simulink library "csu_tcm_thruster_command_metering_lib"  (R2014b)
settings: Solver=ode45  StartTime=0.0  StopTime=10.0  RelTol=1e-3
values from neighbouring files (symbols this model uses):
  act_full_on_duration = uint32( 120 )    [csc_act_actuator_manager_init.m]
libraries: util_common_lib x4, simulink x1, util_info_lib x1
settings Model: Creator=escrane  LastModifiedBy=mstewart

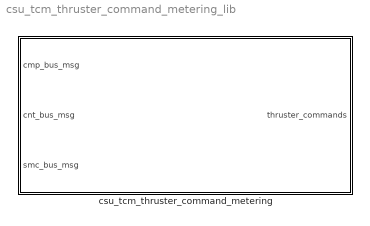
== system csu_tcm_thruster_command_metering_lib ==
  csu_tcm_thruster_command_metering : Subsystem

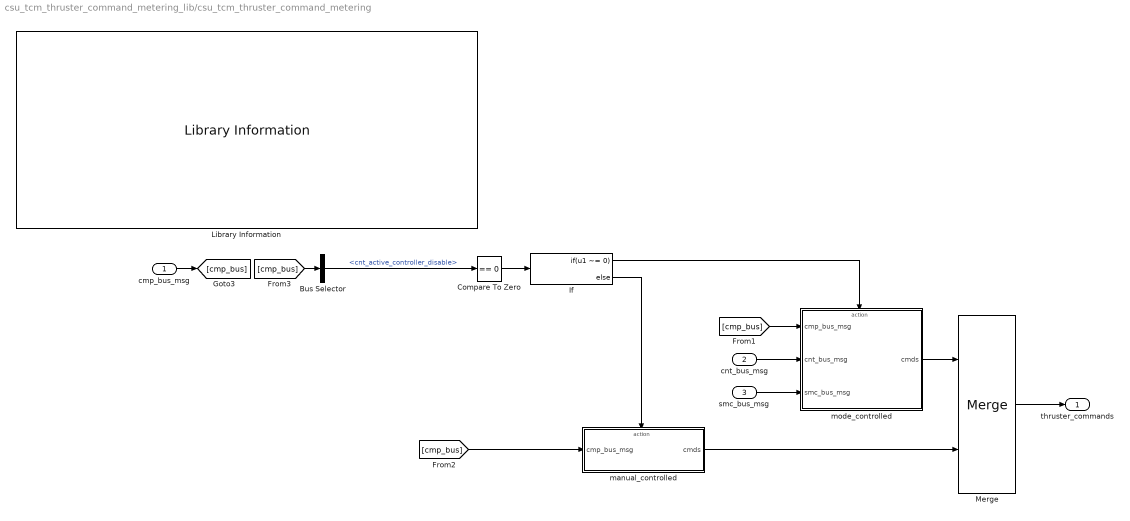
== system csu_tcm_thruster_command_metering_lib/csu_tcm_thruster_command_metering ==
  cmp_bus_msg : Inport
  cnt_bus_msg : Inport  Port=2
  smc_bus_msg : Inport  Port=3
  Bus Selector : BusSelector  OutputSignals=cnt_active_controller_disable
  Compare To Zero : simulink/Logic and Bit Operations/Compare To Zero  relop===  OutDataTypeStr=boolean
  If : If  IfExpression=u1 ~= 0
  Library Information : util_info_lib/Library Information  owner='escrane'
  Merge : Merge
  manual_controlled : Subsystem  TreatAsAtomicUnit=on
  mode_controlled : Subsystem  TreatAsAtomicUnit=on
  thruster_commands : Outport
  wires:
  [cmp_bus] -> manual_controlled/1(cmp_bus_msg)
  If/2 -> manual_controlled/Action
  If/1 -> mode_controlled/Action
  Compare To Zero/1 -> If/1
  [cmp_bus] -> mode_controlled/1(cmp_bus_msg)
  cnt_bus_msg/1 -> mode_controlled/2(cnt_bus_msg)
  smc_bus_msg/1 -> mode_controlled/3(smc_bus_msg)
  [cmp_bus] -> Bus Selector/1
  cmp_bus_msg/1 -> [cmp_bus]
  Merge/1 -> thruster_commands/1
  manual_controlled/1(cmds) -> Merge/2
  mode_controlled/1(cmds) -> Merge/1
  Bus Selector/1 -> Compare To Zero/1  "<cnt_active_controller_disable>"

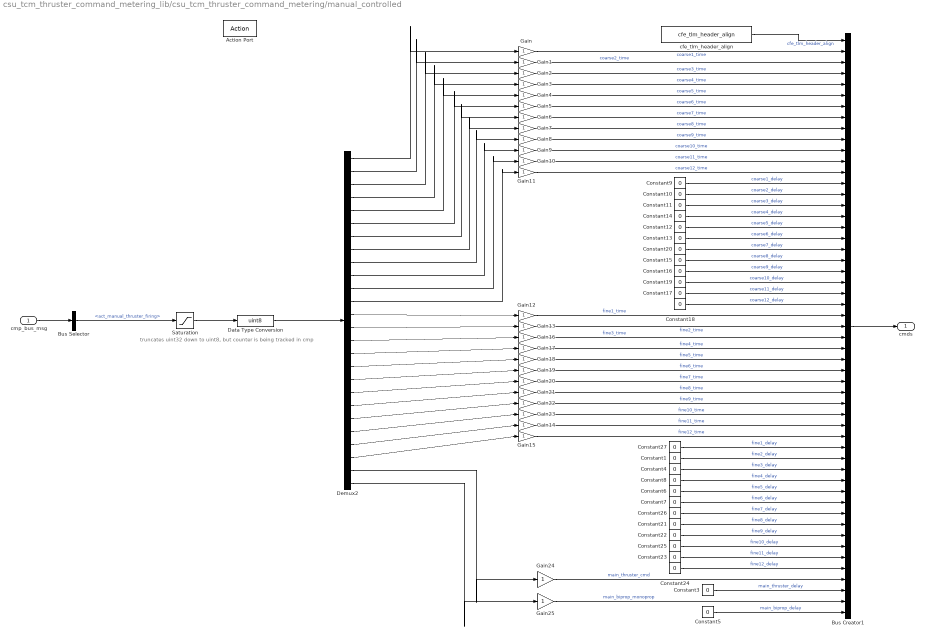
== system csu_tcm_thruster_command_metering_lib/csu_tcm_thruster_command_metering/manual_controlled ==
  note: truncates uint32 down to uint8, but counter is being tracked in cmp
  cmp_bus_msg : Inport
  Action Port : ActionPort
  Bus Creator1 : BusCreator  Inputs=53
  Bus Selector : BusSelector  OutputSignals=act_manual_thruster_firing
  Constant{1,3..27} (26 alike) : Constant  Value=0  OutDataTypeStr=uint8
  Data Type Conversion : DataTypeConversion  OutDataTypeStr=uint8
  Demux2 : Demux  Outputs=26
  Gain{,1..25} (26 alike) : Gain  OutDataTypeStr=uint8
  Saturation : Saturate  UpperLimit=act_full_on_duration  LowerLimit=0
  cfe_tlm_header_align : util_common_lib/cfe_tlm_header_align
  cmds : Outport
  wires:
  Data Type Conversion/1 -> Demux2/1
  Demux2/24 -> Gain15/1
  Demux2/23 -> Gain14/1
  Demux2/22 -> Gain23/1
  Demux2/21 -> Gain22/1
  Demux2/20 -> Gain21/1
  Demux2/19 -> Gain20/1
  Demux2/18 -> Gain19/1
  Demux2/17 -> Gain18/1
  Demux2/16 -> Gain17/1
  Demux2/15 -> Gain16/1
  Demux2/13 -> Gain12/1
  Gain18/1 -> Bus Creator1/30  "fine5_time"
  Gain17/1 -> Bus Creator1/29  "fine4_time"
  Gain13/1 -> Bus Creator1/27  "fine2_time"
  Gain16/1 -> Bus Creator1/28  "fine3_time"
  Demux2/1 -> Gain/1
  Demux2/2 -> Gain1/1
  Demux2/3 -> Gain2/1
  Demux2/4 -> Gain3/1
  Demux2/5 -> Gain4/1
  Demux2/6 -> Gain5/1
  Demux2/12 -> Gain11/1
  Demux2/11 -> Gain10/1
  Demux2/10 -> Gain9/1
  Demux2/9 -> Gain8/1
  Demux2/26 -> Gain25/1
  Demux2/25 -> Gain24/1
  Demux2/8 -> Gain7/1
  Demux2/7 -> Gain6/1
  Bus Selector/1 -> Saturation/1  "<act_manual_thruster_firing>"
  cmp_bus_msg/1 -> Bus Selector/1
  Gain25/1 -> Bus Creator1/52  "main_biprop_monoprop"
  Gain24/1 -> Bus Creator1/50  "main_thruster_cmd"
  Gain3/1 -> Bus Creator1/5  "coarse4_time"
  Bus Creator1/1 -> cmds/1
  cfe_tlm_header_align/1 -> Bus Creator1/1  "cfe_tlm_header_align"
  Gain/1 -> Bus Creator1/2  "coarse1_time"
  Gain7/1 -> Bus Creator1/9  "coarse8_time"
  Gain8/1 -> Bus Creator1/10  "coarse9_time"
  Gain11/1 -> Bus Creator1/13  "coarse12_time"
  Gain6/1 -> Bus Creator1/8  "coarse7_time"
  Gain5/1 -> Bus Creator1/7  "coarse6_time"
  Gain2/1 -> Bus Creator1/4  "coarse3_time"
  Gain4/1 -> Bus Creator1/6  "coarse5_time"
  Gain9/1 -> Bus Creator1/11  "coarse10_time"
  Gain1/1 -> Bus Creator1/3  "coarse2_time"
  Gain10/1 -> Bus Creator1/12  "coarse11_time"
  Constant11/1 -> Bus Creator1/16  "coarse3_delay"
  Constant14/1 -> Bus Creator1/17  "coarse4_delay"
  Constant13/1 -> Bus Creator1/19  "coarse6_delay"
  Constant15/1 -> Bus Creator1/21  "coarse8_delay"
  Constant10/1 -> Bus Creator1/15  "coarse2_delay"
  Constant18/1 -> Bus Creator1/25  "coarse12_delay"
  Constant16/1 -> Bus Creator1/22  "coarse9_delay"
  Constant12/1 -> Bus Creator1/18  "coarse5_delay"
  Constant9/1 -> Bus Creator1/14  "coarse1_delay"
  Constant17/1 -> Bus Creator1/24  "coarse11_delay"
  Constant20/1 -> Bus Creator1/20  "coarse7_delay"
  Constant19/1 -> Bus Creator1/23  "coarse10_delay"
  Gain22/1 -> Bus Creator1/34  "fine9_time"
  Gain23/1 -> Bus Creator1/35  "fine10_time"
  Gain21/1 -> Bus Creator1/33  "fine8_time"
  Gain20/1 -> Bus Creator1/32  "fine7_time"
  Demux2/14 -> Gain13/1
  Gain12/1 -> Bus Creator1/26  "fine1_time"
  Gain15/1 -> Bus Creator1/37  "fine12_time"
  Gain19/1 -> Bus Creator1/31  "fine6_time"
  Gain14/1 -> Bus Creator1/36  "fine11_time"
  Constant5/1 -> Bus Creator1/53  "main_biprop_delay"
  Constant3/1 -> Bus Creator1/51  "main_thruster_delay"
  Constant27/1 -> Bus Creator1/38  "fine1_delay"
  Constant25/1 -> Bus Creator1/47  "fine10_delay"
  Constant8/1 -> Bus Creator1/41  "fine4_delay"
  Constant22/1 -> Bus Creator1/46  "fine9_delay"
  Constant7/1 -> Bus Creator1/43  "fine6_delay"
  Constant4/1 -> Bus Creator1/40  "fine3_delay"
  Constant21/1 -> Bus Creator1/45  "fine8_delay"
  Constant6/1 -> Bus Creator1/42  "fine5_delay"
  Constant1/1 -> Bus Creator1/39  "fine2_delay"
  Constant24/1 -> Bus Creator1/49  "fine12_delay"
  Constant26/1 -> Bus Creator1/44  "fine7_delay"
  Constant23/1 -> Bus Creator1/48  "fine11_delay"
  Saturation/1 -> Data Type Conversion/1

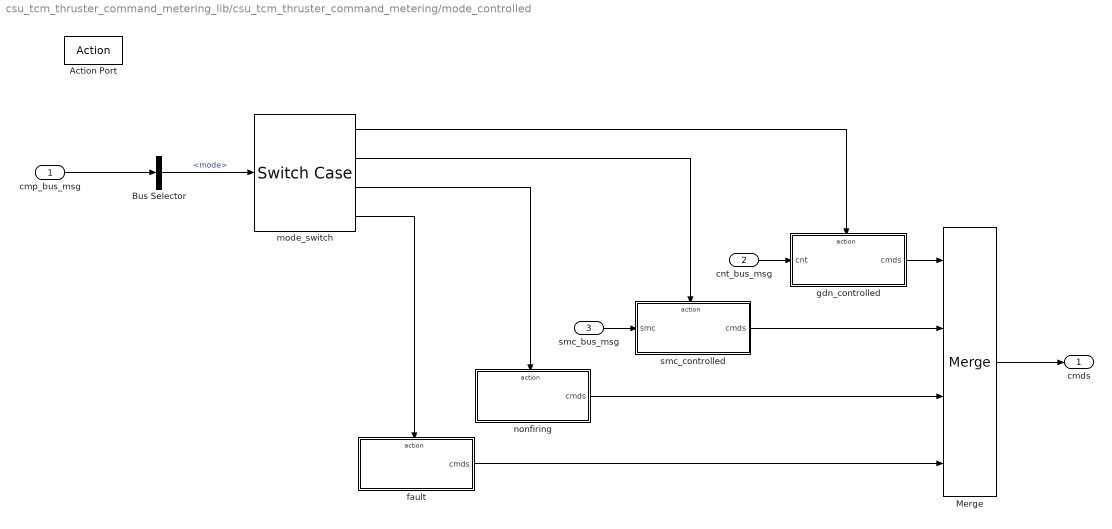
== system csu_tcm_thruster_command_metering_lib/csu_tcm_thruster_command_metering/mode_controlled ==
  cmp_bus_msg : Inport
  cnt_bus_msg : Inport  Port=2
  smc_bus_msg : Inport  Port=3
  Action Port : ActionPort
  Bus Selector : BusSelector  OutputSignals=mode
  Merge : Merge  Inputs=4
  fault : Subsystem  TreatAsAtomicUnit=on
  gdn_controlled : Subsystem  TreatAsAtomicUnit=on
  mode_switch : SwitchCase  CaseConditions={ [uint8(enum_mode.pointing), uint8(enum_mode.deltav), uint8(enum_mode.deorbit), uint8(enum_mode.braking) uint8(enum_mode.landing)], uint8(enum_mode.safe), [uint8(enum_mode.startup), uint8(enum_mode.surface), uint8(enum_mode.safesurface)]}
  nonfiring : Subsystem  TreatAsAtomicUnit=on
  smc_controlled : Subsystem  TreatAsAtomicUnit=on
  cmds : Outport
  wires:
  cmp_bus_msg/1 -> Bus Selector/1
  fault/1(cmds) -> Merge/4
  mode_switch/4 -> fault/Action
  Merge/1 -> cmds/1
  smc_bus_msg/1 -> smc_controlled/1(smc)
  nonfiring/1(cmds) -> Merge/3
  smc_controlled/1(cmds) -> Merge/2
  gdn_controlled/1(cmds) -> Merge/1
  mode_switch/3 -> nonfiring/Action
  mode_switch/2 -> smc_controlled/Action
  mode_switch/1 -> gdn_controlled/Action
  cnt_bus_msg/1 -> gdn_controlled/1(cnt)
  Bus Selector/1 -> mode_switch/1  "<mode>"

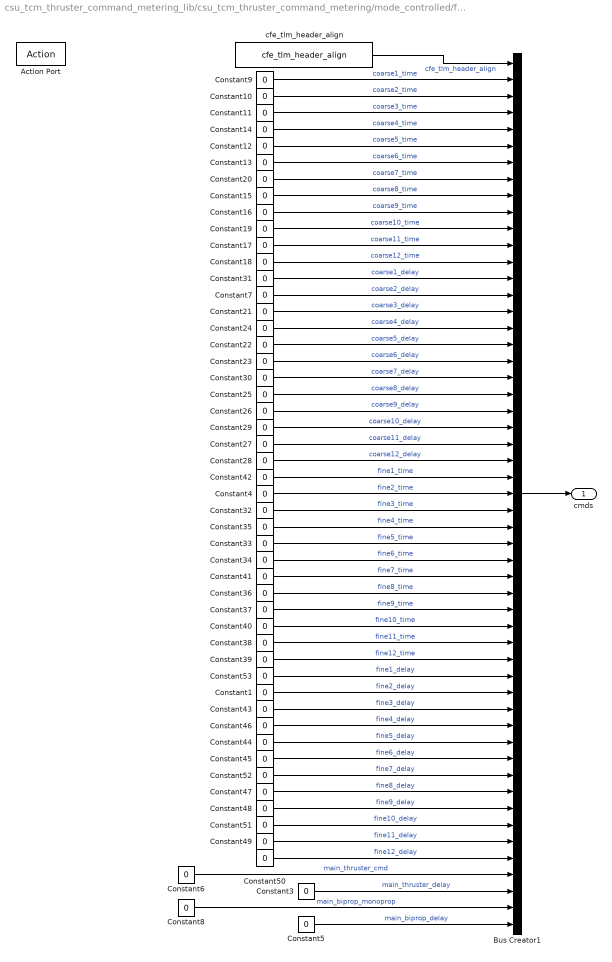
== system csu_tcm_thruster_command_metering_lib/csu_tcm_thruster_command_metering/mode_controlled/fault ==
  Action Port : ActionPort
  Bus Creator1 : BusCreator  Inputs=53
  Constant{1,3..53} (52 alike) : Constant  Value=0  OutDataTypeStr=uint8
  cfe_tlm_header_align : util_common_lib/cfe_tlm_header_align
  cmds : Outport
  wires:
  Bus Creator1/1 -> cmds/1
  Constant8/1 -> Bus Creator1/52  "main_biprop_monoprop"
  Constant6/1 -> Bus Creator1/50  "main_thruster_cmd"
  cfe_tlm_header_align/1 -> Bus Creator1/1  "cfe_tlm_header_align"
  Constant9/1 -> Bus Creator1/2  "coarse1_time"
  Constant15/1 -> Bus Creator1/9  "coarse8_time"
  Constant16/1 -> Bus Creator1/10  "coarse9_time"
  Constant18/1 -> Bus Creator1/13  "coarse12_time"
  Constant20/1 -> Bus Creator1/8  "coarse7_time"
  Constant14/1 -> Bus Creator1/5  "coarse4_time"
  Constant13/1 -> Bus Creator1/7  "coarse6_time"
  Constant11/1 -> Bus Creator1/4  "coarse3_time"
  Constant12/1 -> Bus Creator1/6  "coarse5_time"
  Constant19/1 -> Bus Creator1/11  "coarse10_time"
  Constant10/1 -> Bus Creator1/3  "coarse2_time"
  Constant17/1 -> Bus Creator1/12  "coarse11_time"
  Constant21/1 -> Bus Creator1/16  "coarse3_delay"
  Constant24/1 -> Bus Creator1/17  "coarse4_delay"
  Constant23/1 -> Bus Creator1/19  "coarse6_delay"
  Constant25/1 -> Bus Creator1/21  "coarse8_delay"
  Constant7/1 -> Bus Creator1/15  "coarse2_delay"
  Constant28/1 -> Bus Creator1/25  "coarse12_delay"
  Constant26/1 -> Bus Creator1/22  "coarse9_delay"
  Constant22/1 -> Bus Creator1/18  "coarse5_delay"
  Constant31/1 -> Bus Creator1/14  "coarse1_delay"
  Constant27/1 -> Bus Creator1/24  "coarse11_delay"
  Constant30/1 -> Bus Creator1/20  "coarse7_delay"
  Constant29/1 -> Bus Creator1/23  "coarse10_delay"
  Constant35/1 -> Bus Creator1/29  "fine4_time"
  Constant37/1 -> Bus Creator1/34  "fine9_time"
  Constant40/1 -> Bus Creator1/35  "fine10_time"
  Constant36/1 -> Bus Creator1/33  "fine8_time"
  Constant41/1 -> Bus Creator1/32  "fine7_time"
  Constant4/1 -> Bus Creator1/27  "fine2_time"
  Constant42/1 -> Bus Creator1/26  "fine1_time"
  Constant33/1 -> Bus Creator1/30  "fine5_time"
  Constant39/1 -> Bus Creator1/37  "fine12_time"
  Constant32/1 -> Bus Creator1/28  "fine3_time"
  Constant34/1 -> Bus Creator1/31  "fine6_time"
  Constant38/1 -> Bus Creator1/36  "fine11_time"
  Constant5/1 -> Bus Creator1/53  "main_biprop_delay"
  Constant3/1 -> Bus Creator1/51  "main_thruster_delay"
  Constant53/1 -> Bus Creator1/38  "fine1_delay"
  Constant51/1 -> Bus Creator1/47  "fine10_delay"
  Constant46/1 -> Bus Creator1/41  "fine4_delay"
  Constant48/1 -> Bus Creator1/46  "fine9_delay"
  Constant45/1 -> Bus Creator1/43  "fine6_delay"
  Constant43/1 -> Bus Creator1/40  "fine3_delay"
  Constant47/1 -> Bus Creator1/45  "fine8_delay"
  Constant44/1 -> Bus Creator1/42  "fine5_delay"
  Constant1/1 -> Bus Creator1/39  "fine2_delay"
  Constant50/1 -> Bus Creator1/49  "fine12_delay"
  Constant52/1 -> Bus Creator1/44  "fine7_delay"
  Constant49/1 -> Bus Creator1/48  "fine11_delay"

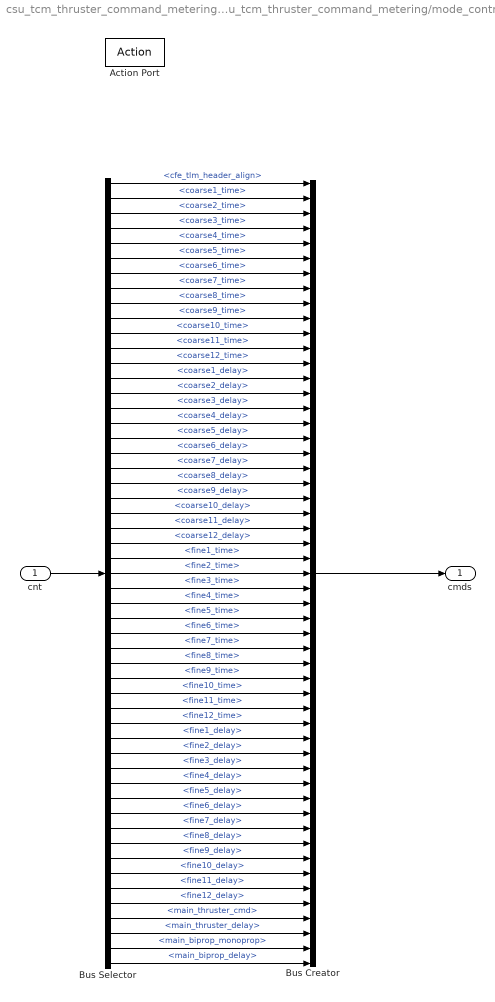
== system csu_tcm_thruster_command_metering_lib/csu_tcm_thruster_command_metering/mode_controlled/gdn_controlled ==
  cnt : Inport
  Action Port : ActionPort
  Bus Creator : BusCreator  Inputs=53
  Bus Selector : BusSelector  OutputSignals=cfe_tlm_header_align,coarse1_time,coarse2_time,coarse3_time,coarse4_time,coarse5_time,coarse6_time,coarse7_time,coarse8_time,coarse9_time,coarse10_time,coarse11_time,coarse12_time,coarse1_delay,coarse2_delay,coarse3_delay,coarse4_delay,coarse5_delay,coarse6_delay,coarse7_delay,coarse8_delay,coarse9_delay,coarse10_delay,coarse11_delay,coarse12_delay,fine1_time,fine2_time,fine3_time,fine4_time,fine5_time,fine6_time,fine7_time,fine8_time,fine9_time,fine10_time,fine11_time,fine12_time,fine1_delay,fine2_delay,fine3_delay,fine4_delay,fine5_delay,fine6_delay,fine7_delay,fine8_delay,fine9_delay,fine10_delay,fine11_delay,fine12_delay,main_thruster_cmd,main_thruster_delay,main_biprop_monoprop,main_biprop_delay
  cmds : Outport
  wires:
  Bus Creator/1 -> cmds/1
  Bus Selector/39 -> Bus Creator/39  "<fine2_delay>"
  Bus Selector/3 -> Bus Creator/3  "<coarse2_time>"
  Bus Selector/27 -> Bus Creator/27  "<fine2_time>"
  Bus Selector/7 -> Bus Creator/7  "<coarse6_time>"
  Bus Selector/50 -> Bus Creator/50  "<main_thruster_cmd>"
  Bus Selector/1 -> Bus Creator/1  "<cfe_tlm_header_align>"
  Bus Selector/18 -> Bus Creator/18  "<coarse5_delay>"
  Bus Selector/42 -> Bus Creator/42  "<fine5_delay>"
  Bus Selector/17 -> Bus Creator/17  "<coarse4_delay>"
  Bus Selector/11 -> Bus Creator/11  "<coarse10_time>"
  Bus Selector/40 -> Bus Creator/40  "<fine3_delay>"
  Bus Selector/10 -> Bus Creator/10  "<coarse9_time>"
  Bus Selector/43 -> Bus Creator/43  "<fine6_delay>"
  Bus Selector/9 -> Bus Creator/9  "<coarse8_time>"
  Bus Selector/28 -> Bus Creator/28  "<fine3_time>"
  Bus Selector/35 -> Bus Creator/35  "<fine10_time>"
  Bus Selector/51 -> Bus Creator/51  "<main_thruster_delay>"
  Bus Selector/37 -> Bus Creator/37  "<fine12_time>"
  Bus Selector/13 -> Bus Creator/13  "<coarse12_time>"
  Bus Selector/21 -> Bus Creator/21  "<coarse8_delay>"
  Bus Selector/38 -> Bus Creator/38  "<fine1_delay>"
  Bus Selector/31 -> Bus Creator/31  "<fine6_time>"
  Bus Selector/6 -> Bus Creator/6  "<coarse5_time>"
  Bus Selector/24 -> Bus Creator/24  "<coarse11_delay>"
  Bus Selector/4 -> Bus Creator/4  "<coarse3_time>"
  Bus Selector/12 -> Bus Creator/12  "<coarse11_time>"
  Bus Selector/23 -> Bus Creator/23  "<coarse10_delay>"
  Bus Selector/33 -> Bus Creator/33  "<fine8_time>"
  Bus Selector/22 -> Bus Creator/22  "<coarse9_delay>"
  Bus Selector/44 -> Bus Creator/44  "<fine7_delay>"
  Bus Selector/45 -> Bus Creator/45  "<fine8_delay>"
  Bus Selector/20 -> Bus Creator/20  "<coarse7_delay>"
  Bus Selector/47 -> Bus Creator/47  "<fine10_delay>"
  Bus Selector/16 -> Bus Creator/16  "<coarse3_delay>"
  Bus Selector/53 -> Bus Creator/53  "<main_biprop_delay>"
  Bus Selector/34 -> Bus Creator/34  "<fine9_time>"
  Bus Selector/49 -> Bus Creator/49  "<fine12_delay>"
  Bus Selector/5 -> Bus Creator/5  "<coarse4_time>"
  Bus Selector/26 -> Bus Creator/26  "<fine1_time>"
  Bus Selector/48 -> Bus Creator/48  "<fine11_delay>"
  Bus Selector/8 -> Bus Creator/8  "<coarse7_time>"
  Bus Selector/52 -> Bus Creator/52  "<main_biprop_monoprop>"
  Bus Selector/46 -> Bus Creator/46  "<fine9_delay>"
  Bus Selector/32 -> Bus Creator/32  "<fine7_time>"
  Bus Selector/19 -> Bus Creator/19  "<coarse6_delay>"
  Bus Selector/2 -> Bus Creator/2  "<coarse1_time>"
  Bus Selector/25 -> Bus Creator/25  "<coarse12_delay>"
  Bus Selector/30 -> Bus Creator/30  "<fine5_time>"
  Bus Selector/36 -> Bus Creator/36  "<fine11_time>"
  Bus Selector/14 -> Bus Creator/14  "<coarse1_delay>"
  Bus Selector/41 -> Bus Creator/41  "<fine4_delay>"
  Bus Selector/15 -> Bus Creator/15  "<coarse2_delay>"
  Bus Selector/29 -> Bus Creator/29  "<fine4_time>"
  cnt/1 -> Bus Selector/1

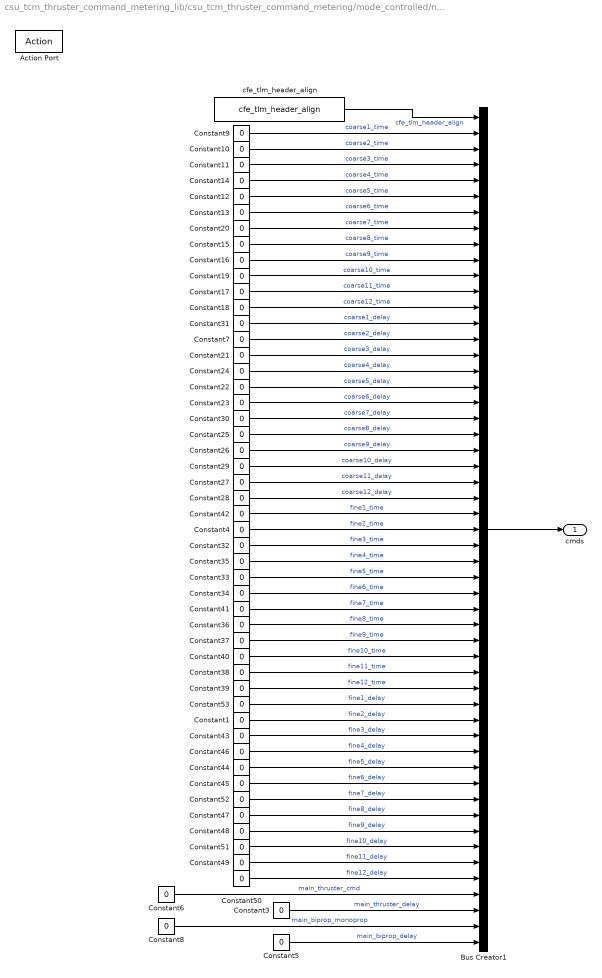
== system csu_tcm_thruster_command_metering_lib/csu_tcm_thruster_command_metering/mode_controlled/nonfiring ==
  Action Port : ActionPort
  Bus Creator1 : BusCreator  Inputs=53
  Constant{1,3..53} (52 alike) : Constant  Value=0  OutDataTypeStr=uint8
  cfe_tlm_header_align : util_common_lib/cfe_tlm_header_align
  cmds : Outport
  wires:
  Constant8/1 -> Bus Creator1/52  "main_biprop_monoprop"
  Constant6/1 -> Bus Creator1/50  "main_thruster_cmd"
  cfe_tlm_header_align/1 -> Bus Creator1/1  "cfe_tlm_header_align"
  Constant9/1 -> Bus Creator1/2  "coarse1_time"
  Constant15/1 -> Bus Creator1/9  "coarse8_time"
  Constant16/1 -> Bus Creator1/10  "coarse9_time"
  Constant18/1 -> Bus Creator1/13  "coarse12_time"
  Constant20/1 -> Bus Creator1/8  "coarse7_time"
  Constant14/1 -> Bus Creator1/5  "coarse4_time"
  Constant13/1 -> Bus Creator1/7  "coarse6_time"
  Constant11/1 -> Bus Creator1/4  "coarse3_time"
  Constant12/1 -> Bus Creator1/6  "coarse5_time"
  Constant19/1 -> Bus Creator1/11  "coarse10_time"
  Constant10/1 -> Bus Creator1/3  "coarse2_time"
  Constant17/1 -> Bus Creator1/12  "coarse11_time"
  Constant21/1 -> Bus Creator1/16  "coarse3_delay"
  Constant24/1 -> Bus Creator1/17  "coarse4_delay"
  Constant23/1 -> Bus Creator1/19  "coarse6_delay"
  Constant25/1 -> Bus Creator1/21  "coarse8_delay"
  Constant7/1 -> Bus Creator1/15  "coarse2_delay"
  Constant28/1 -> Bus Creator1/25  "coarse12_delay"
  Constant26/1 -> Bus Creator1/22  "coarse9_delay"
  Constant22/1 -> Bus Creator1/18  "coarse5_delay"
  Constant31/1 -> Bus Creator1/14  "coarse1_delay"
  Constant27/1 -> Bus Creator1/24  "coarse11_delay"
  Constant30/1 -> Bus Creator1/20  "coarse7_delay"
  Constant29/1 -> Bus Creator1/23  "coarse10_delay"
  Constant35/1 -> Bus Creator1/29  "fine4_time"
  Constant37/1 -> Bus Creator1/34  "fine9_time"
  Constant40/1 -> Bus Creator1/35  "fine10_time"
  Constant36/1 -> Bus Creator1/33  "fine8_time"
  Constant41/1 -> Bus Creator1/32  "fine7_time"
  Constant4/1 -> Bus Creator1/27  "fine2_time"
  Constant42/1 -> Bus Creator1/26  "fine1_time"
  Constant33/1 -> Bus Creator1/30  "fine5_time"
  Constant39/1 -> Bus Creator1/37  "fine12_time"
  Constant32/1 -> Bus Creator1/28  "fine3_time"
  Constant34/1 -> Bus Creator1/31  "fine6_time"
  Constant38/1 -> Bus Creator1/36  "fine11_time"
  Constant5/1 -> Bus Creator1/53  "main_biprop_delay"
  Constant3/1 -> Bus Creator1/51  "main_thruster_delay"
  Constant53/1 -> Bus Creator1/38  "fine1_delay"
  Constant51/1 -> Bus Creator1/47  "fine10_delay"
  Constant46/1 -> Bus Creator1/41  "fine4_delay"
  Constant48/1 -> Bus Creator1/46  "fine9_delay"
  Constant45/1 -> Bus Creator1/43  "fine6_delay"
  Constant43/1 -> Bus Creator1/40  "fine3_delay"
  Constant47/1 -> Bus Creator1/45  "fine8_delay"
  Constant44/1 -> Bus Creator1/42  "fine5_delay"
  Constant1/1 -> Bus Creator1/39  "fine2_delay"
  Constant50/1 -> Bus Creator1/49  "fine12_delay"
  Constant52/1 -> Bus Creator1/44  "fine7_delay"
  Constant49/1 -> Bus Creator1/48  "fine11_delay"
  Bus Creator1/1 -> cmds/1

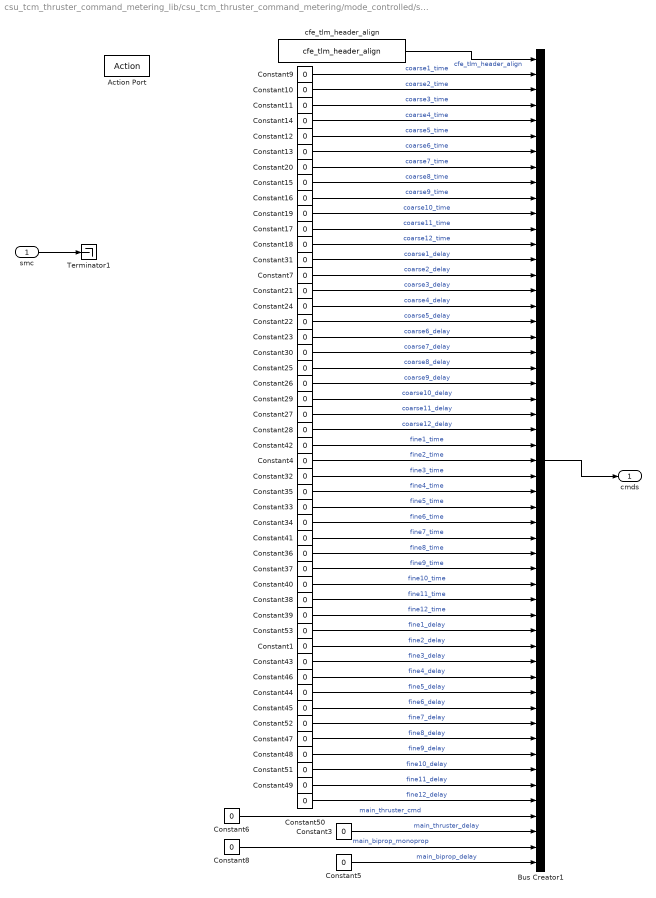
== system csu_tcm_thruster_command_metering_lib/csu_tcm_thruster_command_metering/mode_controlled/smc_controlled ==
  smc : Inport
  Action Port : ActionPort
  Bus Creator1 : BusCreator  Inputs=53
  Constant{1,3..53} (52 alike) : Constant  Value=0  OutDataTypeStr=uint8
  Terminator1 : Terminator
  cfe_tlm_header_align : util_common_lib/cfe_tlm_header_align
  cmds : Outport
  wires:
  Constant8/1 -> Bus Creator1/52  "main_biprop_monoprop"
  Constant6/1 -> Bus Creator1/50  "main_thruster_cmd"
  cfe_tlm_header_align/1 -> Bus Creator1/1  "cfe_tlm_header_align"
  Constant9/1 -> Bus Creator1/2  "coarse1_time"
  Constant15/1 -> Bus Creator1/9  "coarse8_time"
  Constant16/1 -> Bus Creator1/10  "coarse9_time"
  Constant18/1 -> Bus Creator1/13  "coarse12_time"
  Constant20/1 -> Bus Creator1/8  "coarse7_time"
  Constant14/1 -> Bus Creator1/5  "coarse4_time"
  Constant13/1 -> Bus Creator1/7  "coarse6_time"
  Constant11/1 -> Bus Creator1/4  "coarse3_time"
  Constant12/1 -> Bus Creator1/6  "coarse5_time"
  Constant19/1 -> Bus Creator1/11  "coarse10_time"
  Constant10/1 -> Bus Creator1/3  "coarse2_time"
  Constant17/1 -> Bus Creator1/12  "coarse11_time"
  Constant21/1 -> Bus Creator1/16  "coarse3_delay"
  Constant24/1 -> Bus Creator1/17  "coarse4_delay"
  Constant23/1 -> Bus Creator1/19  "coarse6_delay"
  Constant25/1 -> Bus Creator1/21  "coarse8_delay"
  Constant7/1 -> Bus Creator1/15  "coarse2_delay"
  Constant28/1 -> Bus Creator1/25  "coarse12_delay"
  Constant26/1 -> Bus Creator1/22  "coarse9_delay"
  Constant22/1 -> Bus Creator1/18  "coarse5_delay"
  Constant31/1 -> Bus Creator1/14  "coarse1_delay"
  Constant27/1 -> Bus Creator1/24  "coarse11_delay"
  Constant30/1 -> Bus Creator1/20  "coarse7_delay"
  Constant29/1 -> Bus Creator1/23  "coarse10_delay"
  Constant35/1 -> Bus Creator1/29  "fine4_time"
  Constant37/1 -> Bus Creator1/34  "fine9_time"
  Constant40/1 -> Bus Creator1/35  "fine10_time"
  Constant36/1 -> Bus Creator1/33  "fine8_time"
  Constant41/1 -> Bus Creator1/32  "fine7_time"
  Constant4/1 -> Bus Creator1/27  "fine2_time"
  Constant42/1 -> Bus Creator1/26  "fine1_time"
  Constant33/1 -> Bus Creator1/30  "fine5_time"
  Constant39/1 -> Bus Creator1/37  "fine12_time"
  Constant32/1 -> Bus Creator1/28  "fine3_time"
  Constant34/1 -> Bus Creator1/31  "fine6_time"
  Constant38/1 -> Bus Creator1/36  "fine11_time"
  Constant5/1 -> Bus Creator1/53  "main_biprop_delay"
  Constant3/1 -> Bus Creator1/51  "main_thruster_delay"
  Constant53/1 -> Bus Creator1/38  "fine1_delay"
  Constant51/1 -> Bus Creator1/47  "fine10_delay"
  Constant46/1 -> Bus Creator1/41  "fine4_delay"
  Constant48/1 -> Bus Creator1/46  "fine9_delay"
  Constant45/1 -> Bus Creator1/43  "fine6_delay"
  Constant43/1 -> Bus Creator1/40  "fine3_delay"
  Constant47/1 -> Bus Creator1/45  "fine8_delay"
  Constant44/1 -> Bus Creator1/42  "fine5_delay"
  Constant1/1 -> Bus Creator1/39  "fine2_delay"
  Constant50/1 -> Bus Creator1/49  "fine12_delay"
  Constant52/1 -> Bus Creator1/44  "fine7_delay"
  Constant49/1 -> Bus Creator1/48  "fine11_delay"
  Bus Creator1/1 -> cmds/1
  smc/1 -> Terminator1/1
